simulink model "MuscleSpindleGUIModel"  (Simulink 7.9)
settings: Solver=ode3  StartTime=0.0  StopTime=inf  FixedStep=1e-3  RelTol=1e-3
StartFcn:
  | SetupCallbacks
libraries: simulink x1
settings Model: Creator=oli  LastModifiedBy=oli  BufferReuse=off
settings OptimizationCC: BlockReduction=off  BufferReuse=off
settings DebuggingCC: AlgebraicLoopMsg=none  SolverPrmCheckMsg=none  UnconnectedInputMsg=none  UnconnectedOutputMsg=none  UnconnectedLineMsg=none

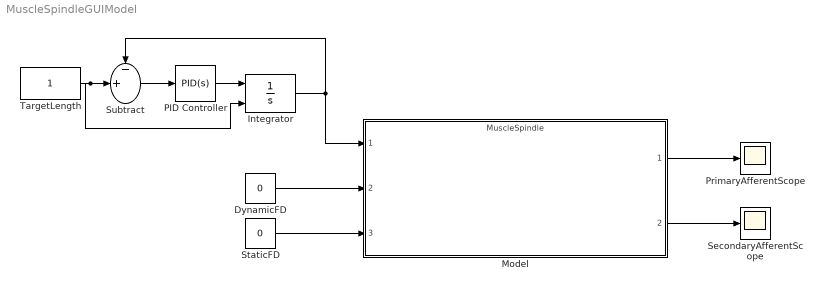
== system MuscleSpindleGUIModel ==
  DynamicFD : Constant  Value=0
  Integrator : Integrator  InitialConditionSource=external
  Model : ModelReference  ModelNameDialog=MuscleSpindle  SimulationMode=Normal  ModelReferenceVersion=1.475  CopyOfModelName=MuscleSpindle  DefaultDataLogging=on
  PID Controller : simulink/Continuous/PID Controller  Controller=PID  TimeDomain=Continuous-time  SampleTime=1  IntegratorMethod=Forward Euler  FilterMethod=Forward Euler  Form=Parallel  P=5  I=0.75  D=0.25  N=100  InitialConditionSource=internal  InitialConditionForIntegrator=0  InitialConditionForFilter=0  ExternalReset=none  LimitOutput=off  UpperSaturationLimit=inf  LowerSaturationLimit=-inf  LinearizeAsGain=off  AntiWindupMode=none  Kb=1  TrackingMode=off  Kt=1  PParamMin=[]  PParamMax=[]  IParamMin=[]  IParamMax=[]  DParamMin=[]  DParamMax=[]  NParamMin=[]  NParamMax=[]  KbParamMin=[]  KbParamMax=[]  KtParamMin=[]  KtParamMax=[]  POutMin=[]  POutMax=[]  IOutMin=[]  IOutMax=[]  DOutMin=[]  DOutMax=[]  NOutMin=[]  NOutMax=[]  KbOutMin=[]  KbOutMax=[]  KtOutMin=[]  KtOutMax=[]  IntegratorOutMin=[]  IntegratorOutMax=[]  FilterOutMin=[]  FilterOutMax=[]  SumOutMin=[]  SumOutMax=[]  SumI1OutMin=[]  SumI1OutMax=[]  SumI2OutMin=[]  SumI2OutMax=[]  SumI3OutMin=[]  SumI3OutMax=[]  SumDOutMin=[]  SumDOutMax=[]  SaturationOutMin=[]  SaturationOutMax=[]  IntegratorContinuousStateAttributes=''  IntegratorStateMustResolveToSignalObject=off  IntegratorRTWStateStorageClass=Auto  FilterContinuousStateAttributes=''  FilterStateMustResolveToSignalObject=off  FilterRTWStateStorageClass=Auto
  PrimaryAfferentScope : Scope
  SecondaryAfferentScope : Scope
  StaticFD : Constant  Value=0
  Subtract : Sum  Inputs=-+|
  TargetLength : Constant
  wires:
  DynamicFD/1 -> Model/2
  StaticFD/1 -> Model/3
  Model/1 -> PrimaryAfferentScope/1
  Model/2 -> SecondaryAfferentScope/1
  PID Controller/1 -> Integrator/1
  TargetLength/1 -> Subtract/2, Integrator/2
  Subtract/1 -> PID Controller/1
  Integrator/1 -> Model/1, Subtract/1
